simulink model "bipolarh4..."  (R2018a)
settings: Solver=VariableStepAuto  StartTime=0.0  StopTime=.1  RelTol=1e-3
libraries: powerlib x19, powerlib_meascontrol x4, simulink x1
settings Model: Creator=Razowan  LastModifiedBy=Razowan

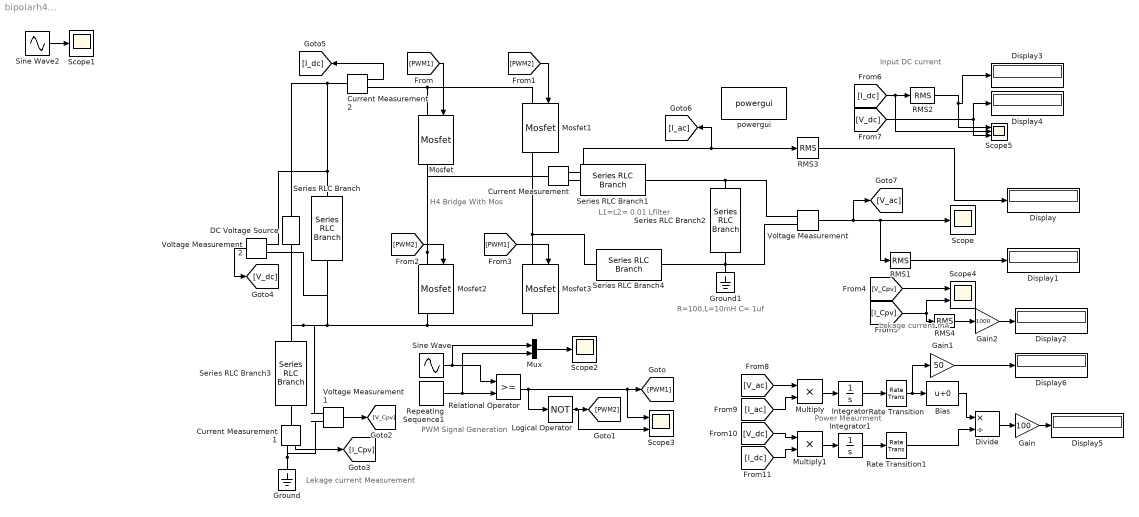
== system bipolarh4... ==
  note: L1=L2= 0.01 Lfilter
  note: H4 Bridge With Mos
  note: Lekage current mA
  note: Power Meaurment
  note: PWM Signal Generation
  note: Input DC current
  note: R=100,L=10mH C= 1uf
  note: Lekage current Measurement
  Bias : Bias
  Current Measurement : powerlib/Measurements/Current Measurement  PhasorSimulation=off  OutputType=Complex  PSBequivalent=0
  Current Measurement1 : powerlib/Measurements/Current Measurement  PhasorSimulation=off  OutputType=Complex  PSBequivalent=0
  Current Measurement2 : powerlib/Measurements/Current Measurement  PhasorSimulation=off  OutputType=Complex  PSBequivalent=0
  DC Voltage Source : powerlib/Electrical Sources/DC Voltage Source  Amplitude=460  Measurements=None
  Display{,1..6} (7 alike) : Display
  Divide : Product  Inputs=*/
  Gain : Gain  Gain=100
  Gain1 : Gain  Gain=50
  Gain2 : Gain  Gain=1000
  Ground : powerlib/Elements/Ground  LConnTagsString=a
  Ground1 : powerlib/Elements/Ground  LConnTagsString=a
  Integrator : Integrator
  Integrator1 : Integrator
  Logical Operator : Logic  Operator=NOT  AllPortsSameDT=off  OutDataTypeStr=boolean
  Mosfet{,1..3} (4 alike) : powerlib/Power Electronics/Mosfet  Ron=0.1  Lon=0  Rd=0.01  Vfd=0  IC=0  Rs=1e5  Cs=inf  Measurements=on
  Multiply : Product
  Multiply1 : Product
  Mux : Mux  Inputs=2
  RMS1 : powerlib_meascontrol/Measurements/RMS  TrueRMS=on  Freq=50  RMSInit=0  Ts=0
  RMS2 : powerlib_meascontrol/Measurements/RMS  TrueRMS=on  Freq=50  RMSInit=0  Ts=0
  RMS3 : powerlib_meascontrol/Measurements/RMS  TrueRMS=on  Freq=60  RMSInit=120  Ts=0
  RMS4 : powerlib_meascontrol/Measurements/RMS  TrueRMS=on  Freq=50  RMSInit=0  Ts=0
  Rate Transition : RateTransition
  Rate Transition1 : RateTransition
  Relational Operator : RelationalOperator  OutDataTypeStr=boolean  RndMeth=Simplest
  Repeating Sequence1 : simulink/Sources/Repeating Sequence  rep_seq_t=[0 1 2 3 4]*[1/10000]  rep_seq_y=[0 1 0 -1 0]
  Scope : Scope
  Scope1 : Scope
  Scope2 : Scope
  Scope3 : Scope  NumInputPorts=2
  Scope4 : Scope  NumInputPorts=2
  Scope5 : Scope  NumInputPorts=3
  Series RLC Branch : powerlib/Elements/Series RLC Branch  LConnTagsString=__new0  RConnTagsString=__new0  BranchType=RC  Resistance=.049  Inductance=1e-3  SetiL0=off  InitialCurrent=0  Capacitance=.94  Setx0=off  InitialVoltage=0  Measurements=None
  Series RLC Branch1 : powerlib/Elements/Series RLC Branch  LConnTagsString=__new0  RConnTagsString=__new0  BranchType=L  Resistance=1  Inductance=.01  SetiL0=off  InitialCurrent=0  Capacitance=1e-6  Setx0=off  InitialVoltage=0  Measurements=None
  Series RLC Branch2 : powerlib/Elements/Series RLC Branch  LConnTagsString=__new0  RConnTagsString=__new0  BranchType=R  Resistance=10  Inductance=10e-3  SetiL0=off  InitialCurrent=0  Capacitance=1e-6  Setx0=off  InitialVoltage=0  Measurements=None
  Series RLC Branch3 : powerlib/Elements/Series RLC Branch  LConnTagsString=__new0  RConnTagsString=__new0  BranchType=C  Resistance=1  Inductance=1e-3  SetiL0=off  InitialCurrent=0  Capacitance=150e-9  Setx0=off  InitialVoltage=0  Measurements=None
  Series RLC Branch4 : powerlib/Elements/Series RLC Branch  LConnTagsString=__new0  RConnTagsString=__new0  BranchType=L  Resistance=1  Inductance=.01  SetiL0=off  InitialCurrent=0  Capacitance=1e-6  Setx0=off  InitialVoltage=0  Measurements=None
  Sine Wave : Sin  Frequency=2*pi*50  SampleTime=0
  Sine Wave2 : Sin  Frequency=2*pi*50  SampleTime=.000001  Offset=5
  Voltage Measurement : powerlib/Measurements/Voltage Measurement  PhasorSimulation=off  OutputType=Complex  PSBequivalent=0
  Voltage Measurement1 : powerlib/Measurements/Voltage Measurement  PhasorSimulation=off  OutputType=Complex  PSBequivalent=0
  Voltage Measurement2 : powerlib/Measurements/Voltage Measurement  PhasorSimulation=off  OutputType=Complex  PSBequivalent=0
  powergui : powerlib/powergui  Priority=1  SimulationMode=Continuous  SampleTime=50e-6  frequency=60  Iterations=50  frequencyindice=0  Pbase=100e6  ErrMax=1e-4  UnitsV=kV  UnitsW=MW  buscounter=0  FunctionMessages=off  echomessages=off  EnableUseOfTLC=off  CurrentSourceSwitches=off  DisableSnubberDevices=off  DisableRonSwitches=off  DisableVfSwitches=off  DisplayEquations=off  SolverType=Tustin/Backward Euler (TBE)  Interpol=off  ExternalGateDelay=off  methode=off  Ts=100  x0status=blocks  SPID=on  SwTol=0  HookPort=off  RestoreLinks=warning  ResistiveCurrentMeasurement=off  Frange=[0:2:500]  Ylog=off  Xlog=on  ShowGrid=off  save=off  variable=ZData  structure=bipolarH4  ZoomFFT=off  StartTime=0.01  cycles=4  DisplayStyle=1  fundamental=50  FreqAxis=on  MaxFrequency=2000  frequencyindicesteady=1  RmsSteady=1  display=off
  wires:
  Repeating Sequence1/1 -> Relational Operator/2, Mux/2
  [PWM1] -> Mosfet/1
  Voltage Measurement/1 -> Scope/1, RMS1/1, [V_ac]
  [PWM2] -> Mosfet2/1
  [PWM2] -> Mosfet1/1
  [PWM1] -> Mosfet3/1
  Sine Wave/1 -> Mux/1, Relational Operator/1
  Mux/1 -> Scope2/1
  Relational Operator/1 -> Scope3/1, [PWM1], Logical Operator/1
  Logical Operator/1 -> Scope3/2, [PWM2]
  Sine Wave2/1 -> Scope1/1
  Current Measurement/1 -> [I_ac], RMS3/1
  RMS3/1 -> Display/1
  RMS1/1 -> Display1/1
  Voltage Measurement1/1 -> [V_Cpv]
  Current Measurement1/1 -> [I_Cpv]
  [I_Cpv] -> RMS4/1, Scope4/2
  [V_Cpv] -> Scope4/1
  Voltage Measurement2/1 -> [V_dc]
  Current Measurement2/1 -> [I_dc]
  [I_dc] -> Scope5/2, RMS2/1
  RMS2/1 -> Scope5/1, Display3/1
  [V_dc] -> Scope5/3, Display4/1
  RMS4/1 -> Gain2/1
  [V_ac] -> Multiply/1
  [I_ac] -> Multiply/2
  [V_dc] -> Multiply1/1
  [I_dc] -> Multiply1/2
  Multiply/1 -> Integrator/1
  Multiply1/1 -> Integrator1/1
  Integrator/1 -> Rate Transition/1
  Integrator1/1 -> Rate Transition1/1
  Rate Transition/1 -> Bias/1, Gain1/1
  Bias/1 -> Divide/1
  Rate Transition1/1 -> Divide/2
  Divide/1 -> Gain/1
  Gain/1 -> Display5/1
  Gain1/1 -> Display6/1
  Gain2/1 -> Display2/1
  connections:
  Mosfet2/RConn1 -- Voltage Measurement2/LConn2 -- Series RLC Branch/RConn1 -- Series RLC Branch3/LConn1 -- DC Voltage Source/LConn1 -- Voltage Measurement1/LConn2 -- Mosfet3/RConn1
  Voltage Measurement/LConn2 -- Ground1/LConn1 -- Series RLC Branch2/RConn1 -- Series RLC Branch4/RConn1
  Voltage Measurement/LConn1 -- Series RLC Branch1/RConn1 -- Series RLC Branch2/LConn1
  Mosfet2/LConn1 -- Mosfet/RConn1 -- Current Measurement/LConn1
  Series RLC Branch/LConn1 -- Voltage Measurement2/LConn1 -- DC Voltage Source/RConn1 -- Current Measurement2/LConn1
  Series RLC Branch3/RConn1 -- Current Measurement1/LConn1
  Ground/LConn1 -- Voltage Measurement1/LConn1 -- Current Measurement1/RConn1
  Mosfet1/RConn1 -- Series RLC Branch4/LConn1 -- Mosfet3/LConn1
  Series RLC Branch1/LConn1 -- Current Measurement/RConn1
  Mosfet1/LConn1 -- Mosfet/LConn1 -- Current Measurement2/RConn1
